simulink model "batModelSimulink"  (R2021a)
settings: Solver=FixedStepAuto  StartTime=0.0  StopTime=endTime  FixedStep=ts  RelTol=1e-3
values from neighbouring files (symbols this model uses):
  alpha = cellModel.alpha    [runBatModelSimulink.m]
  rs = cellModel.rs    [runBatModelSimulink.m]
undefined symbols (not defined in the file or in its folder): denC, denDtc1, numC, numDtc1, vocFitSimulink
settings Model: Creator=Ausgang  LastModifiedBy=Augusto Tavares
settings SolverCC: AlgebraicLoopSolver=TrustRegion
settings DataIOCC: ReturnWorkspaceOutputs=off
settings DebuggingCC: SFMachineParentedDataDiag=warning
settings SFSimCC: CustomCodeUndefinedFunction=UseInterfaceOnly

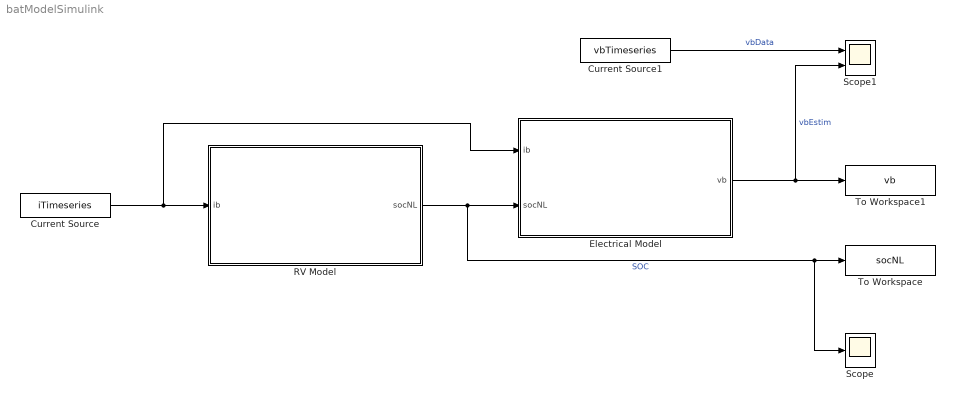
== system batModelSimulink ==
  Current Source : FromWorkspace  VariableName=iTimeseries
  Current Source1 : FromWorkspace  VariableName=vbTimeseries
  Electrical Model : Subsystem
  RV Model : Subsystem
  Scope : Scope
  Scope1 : Scope  NumInputPorts=2
  To Workspace : ToWorkspace  VariableName=socNL  SaveFormat=Timeseries  SampleTime=-1
  To Workspace1 : ToWorkspace  VariableName=vb  SaveFormat=Timeseries  SampleTime=-1
  wires:
  RV Model/1(socNL) -> Scope/1, To Workspace/1, Electrical Model/2(socNL)  "SOC"
  Electrical Model/1(vb) -> To Workspace1/1, Scope1/2  "vbEstim"
  Current Source/1 -> Electrical Model/1(ib), RV Model/1(ib)
  Current Source1/1 -> Scope1/1  "vbData"

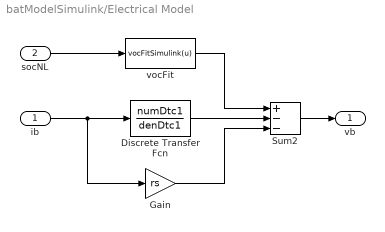
== system batModelSimulink/Electrical Model ==
  ib : Inport
  socNL : Inport  Port=2
  Discrete Transfer Fcn : DiscreteTransferFcn  Numerator=numDtc1  Denominator=denDtc1
  Gain : Gain  Gain=rs
  Sum2 : Sum  Inputs=+--
  vocFit : MATLABFcn  MATLABFcn=vocFitSimulink(u)
  vb : Outport  VectorParamsAs1DForOutWhenUnconnected=off
  wires:
  socNL/1 -> vocFit/1
  vocFit/1 -> Sum2/1
  Sum2/1 -> vb/1
  ib/1 -> Gain/1, Discrete Transfer Fcn/1
  Gain/1 -> Sum2/3
  Discrete Transfer Fcn/1 -> Sum2/2

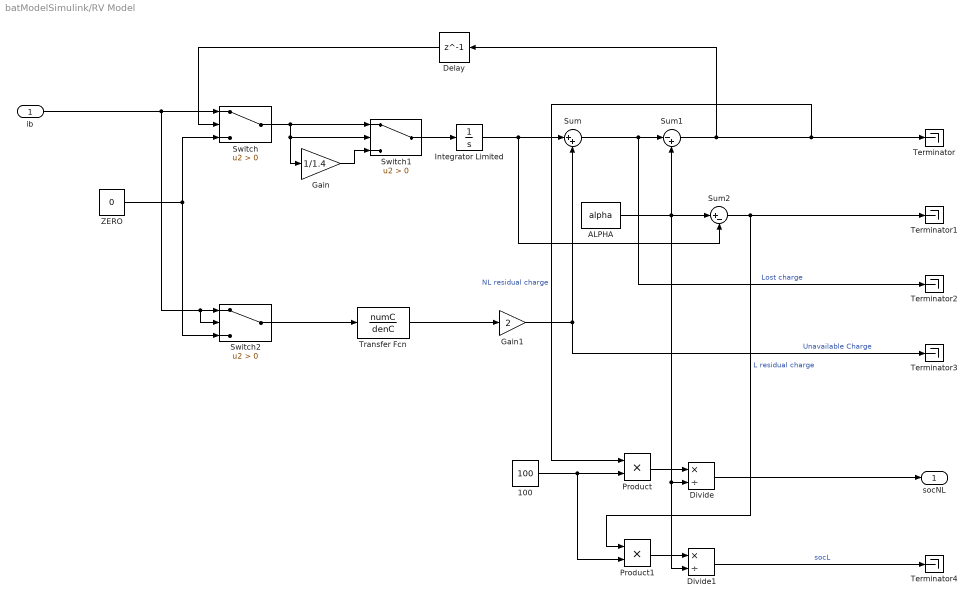
== system batModelSimulink/RV Model ==
  ib : Inport
  100 : Constant  Value=100
  ALPHA : Constant  Value=alpha
  Delay : Delay  DelayLength=1
  Divide : Product  Inputs=*/
  Divide1 : Product  Inputs=*/
  Gain : Gain  Gain=1/1.4
  Gain1 : Gain  Gain=2
  Integrator Limited : Integrator  LimitOutput=on  UpperSaturationLimit=alpha  LowerSaturationLimit=0
  Product : Product
  Product1 : Product
  Sum : Sum  Inputs=|++
  Sum1 : Sum  Inputs=|-+
  Sum2 : Sum  Inputs=|+-
  Switch : Switch  Criteria=u2 > Threshold
  Switch1 : Switch  Criteria=u2 > Threshold
  Switch2 : Switch  Criteria=u2 > Threshold
  Terminator{,1..4} (5 alike) : Terminator
  Transfer Fcn : TransferFcn  Numerator=numC  Denominator=denC
  ZERO : Constant  Value=0
  socNL : Outport  VectorParamsAs1DForOutWhenUnconnected=off
  wires:
  Switch2/1 -> Transfer Fcn/1
  ib/1 -> Switch2/2, Switch2/1, Switch/1
  Switch/1 -> Gain/1, Switch1/2, Switch1/1
  ZERO/1 -> Switch2/3, Switch/3
  Integrator Limited/1 -> Sum/1, Sum2/2
  Sum/1 -> Terminator2/1, Sum1/1  "Lost charge"
  Gain/1 -> Switch1/3
  Delay/1 -> Switch/2
  Switch1/1 -> Integrator Limited/1
  ALPHA/1 -> Sum2/1, Divide1/2, Divide/2, Sum1/2
  Product/1 -> Divide/1
  Divide/1 -> socNL/1
  Sum2/1 -> Terminator1/1, Product1/1  "L residual charge"
  100/1 -> Product1/2, Product/2
  Product1/1 -> Divide1/1
  Divide1/1 -> Terminator4/1  "socL"
  Transfer Fcn/1 -> Gain1/1
  Gain1/1 -> Terminator3/1, Sum/2  "Unavailable Charge"
  Sum1/1 -> Terminator/1, Product/1, Delay/1  "NL residual charge"
